simulink model "fadec_model"  (R2025b)
settings: Solver=FixedStepDiscrete  StartTime=0.0  StopTime=35  FixedStep=0.02  RelTol=1e-3
libraries: simulink x1
settings DataIOCC: InspectSignalLogs=on  LoggingToFile=on

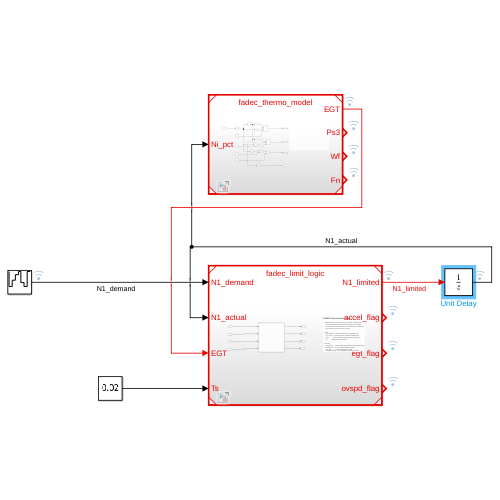
[thumbnail: Simulink's stored preview of the top-level diagram]
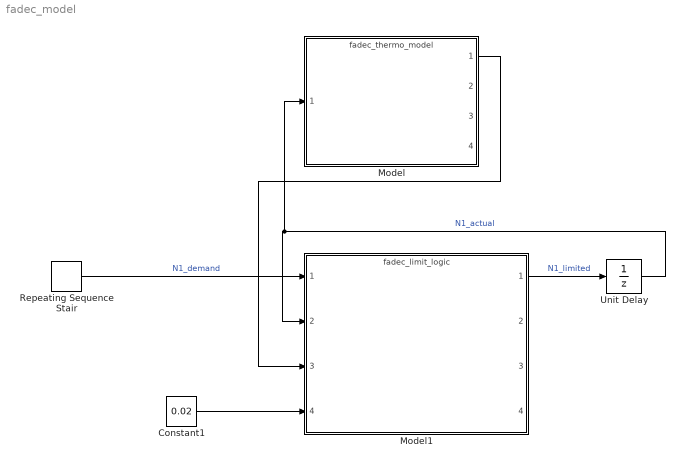
== system fadec_model ==
  Constant1 : Constant  Value=0.02
  Model : ModelReference  ModelNameDialog=fadec_thermo_model.slx  SimulationMode=Normal  ModelReferenceVersion=1.13
  Model1 : ModelReference  ModelNameDialog=fadec_limit_logic.slx  SimulationMode=Normal  ModelReferenceVersion=1.4
  Repeating Sequence Stair : simulink/Sources/Repeating Sequence Stair  OutValues=[19 50 80 95 40 19 95].'  tsamp=[7 5]  OutMin=[]  OutMax=[]  OutDataTypeStr=double  OutputDataTypeScalingMode=double  OutDataType=fixdt(0,8)  ConRadixGroup=Best Precision: Vector-wise  OutScaling=2^-12
  Unit Delay : UnitDelay  InitialCondition=19  SampleTime=-1  HasFrameUpgradeWarning=on
  wires:
  Repeating Sequence Stair/1 -> Model1/1  "N1_demand"
  Model1/1 -> Unit Delay/1  "N1_limited"
  Unit Delay/1 -> Model/1, Model1/2  "N1_actual"
  Model/1 -> Model1/3
  Constant1/1 -> Model1/4
